simulink model "acc_to_v"  (R2015b)
settings: Solver=VariableStepAuto  StartTime=0.0  StopTime=10.0  RelTol=1e-3
undefined symbols (not defined in the file or in its folder): DiscIntNeverNeededParam
libraries: robotlib x2
settings Model: Creator=erik  LastModifiedBy=erik

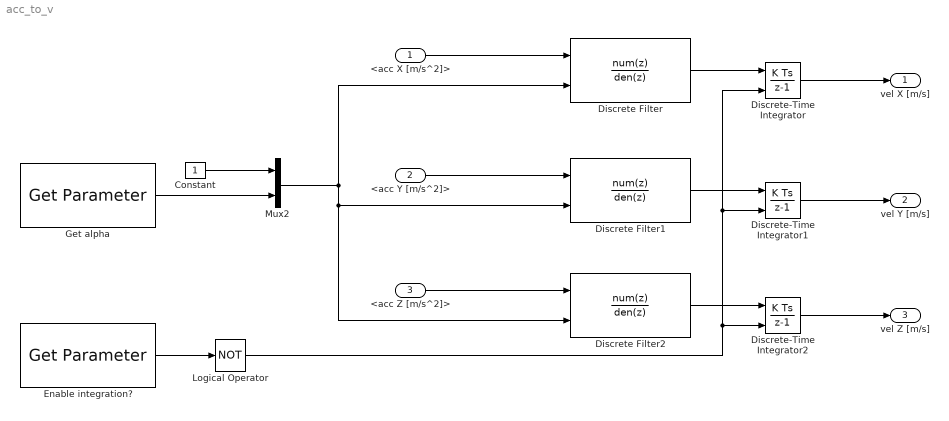
== system acc_to_v ==
  "<acc X [m/s^2]> " : Inport
  <acc Y [m/s^2]> : Inport  Port=2
  <acc Z [m/s^2]> : Inport  Port=3
  Constant : Constant
  Discrete Filter : DiscreteFilter  DenominatorSource=Input port  FilterStructure=Direct form I  a0EqualsOne=on
      settings: InputPortMap=u0,p3
  Discrete Filter1 : DiscreteFilter  DenominatorSource=Input port  FilterStructure=Direct form I  a0EqualsOne=on
      settings: InputPortMap=u0,p3
  Discrete Filter2 : DiscreteFilter  DenominatorSource=Input port  FilterStructure=Direct form I  a0EqualsOne=on
      settings: InputPortMap=u0,p3
  Discrete-Time Integrator : DiscreteIntegrator  ExternalReset=sampled level  InitialConditionSetting=State (most efficient)  SampleTime=-1  ICPrevOutput=DiscIntNeverNeededParam  ICPrevScaledInput=DiscIntNeverNeededParam
  Discrete-Time Integrator1 : DiscreteIntegrator  ExternalReset=sampled level  InitialConditionSetting=State (most efficient)  SampleTime=-1  ICPrevOutput=DiscIntNeverNeededParam  ICPrevScaledInput=DiscIntNeverNeededParam
  Discrete-Time Integrator2 : DiscreteIntegrator  ExternalReset=sampled level  InitialConditionSetting=State (most efficient)  SampleTime=-1  ICPrevOutput=DiscIntNeverNeededParam  ICPrevScaledInput=DiscIntNeverNeededParam
  Enable integration? : robotlib/Get Parameter  SourceLibraryInfo=This block requires Robotics System Toolbox  ParameterSource=Select from ROS network  ParameterName=/matlab_controller/enable_integration  ParameterType=boolean  ParameterInitialValue=0.0  SampleTime=-1  ShowErrorCodeOutput=off  ModelName=Controller_without_ref  BlockId=ParamGet_Controller_without_ref_685
  Get alpha : robotlib/Get Parameter  SourceLibraryInfo=This block requires Robotics System Toolbox  ParameterSource=Select from ROS network  ParameterName=/matlab_controller/alpha  ParameterType=double  ParameterInitialValue=0.0  SampleTime=-1  ShowErrorCodeOutput=off  ModelName=Controller_without_ref  BlockId=ParamGet_Controller_without_ref_672
  Logical Operator : Logic  Operator=NOT  AllPortsSameDT=off  OutDataTypeStr=boolean
  Mux2 : Mux  Inputs=2
  "vel X [m/s] " : Outport
  vel Y [m/s] : Outport  Port=2
  vel Z [m/s] : Outport  Port=3
  wires:
  Discrete-Time Integrator/1 -> "vel X [m/s] "/1
  Discrete-Time Integrator1/1 -> vel Y [m/s]/1
  Discrete-Time Integrator2/1 -> vel Z [m/s]/1
  "<acc X [m/s^2]> "/1 -> Discrete Filter/1
  Discrete Filter/1 -> Discrete-Time Integrator/1
  Discrete Filter1/1 -> Discrete-Time Integrator1/1
  Discrete Filter2/1 -> Discrete-Time Integrator2/1
  <acc Z [m/s^2]>/1 -> Discrete Filter2/1
  <acc Y [m/s^2]>/1 -> Discrete Filter1/1
  Mux2/1 -> Discrete Filter2/2, Discrete Filter1/2, Discrete Filter/2
  Get alpha/1 -> Mux2/2
  Constant/1 -> Mux2/1
  Enable integration?/1 -> Logical Operator/1
  Logical Operator/1 -> Discrete-Time Integrator/2, Discrete-Time Integrator1/2, Discrete-Time Integrator2/2
